simulink model "ball_and_beam"  (R2023b)
settings: Solver=VariableStepAuto  StartTime=0.0  StopTime=inf  RelTol=1e-3
values from neighbouring files (symbols this model uses):
  A = [0  1; 0  0]    [1-dof.mat]    (also in 2-dof.mat = [0 0 0 0 1 0 0 0 0 0 0 0 ... (16 elements, 4x4)]; ball_balancing_platform.mat = [0 0 0 0 0 0 0 0 0 0 0 0 ... (64 elements, 8x8)])
  B = [0 -0.1692]    [1-dof.mat]    (also in 2-dof.mat = [0  0; -0.253868468945  0; 0  0; 0  0.253868468945]; ball_balancing_platform.mat = [0 0 0 0 0 0 1 0 0 0 0 0 ... (16 elements, 8x2)])
  C = [1 0]    [1-dof.mat]    (also in 2-dof.mat = [1  0  0  0; 0  0  1  0]; ball_balancing_platform.mat = [1 0 0 0 0 1 0 0 0 0 1 0 ... (32 elements, 4x8)])
  D = 0    [1-dof.mat]    (also in 2-dof.mat = [0  0; 0  0]; ball_balancing_platform.mat = [0  0; 0  0; 0  0; 0  0])
libraries: robotlib x2, mpclib x1, aerolibanimutils x1
settings Model: Creator=farhan  LastModifiedBy=farhan

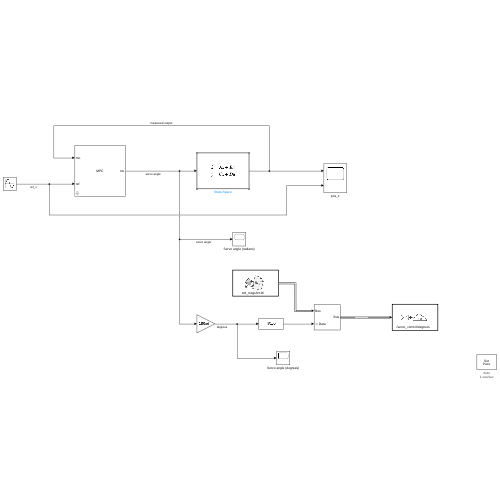
[thumbnail: Simulink's stored preview of the top-level diagram]
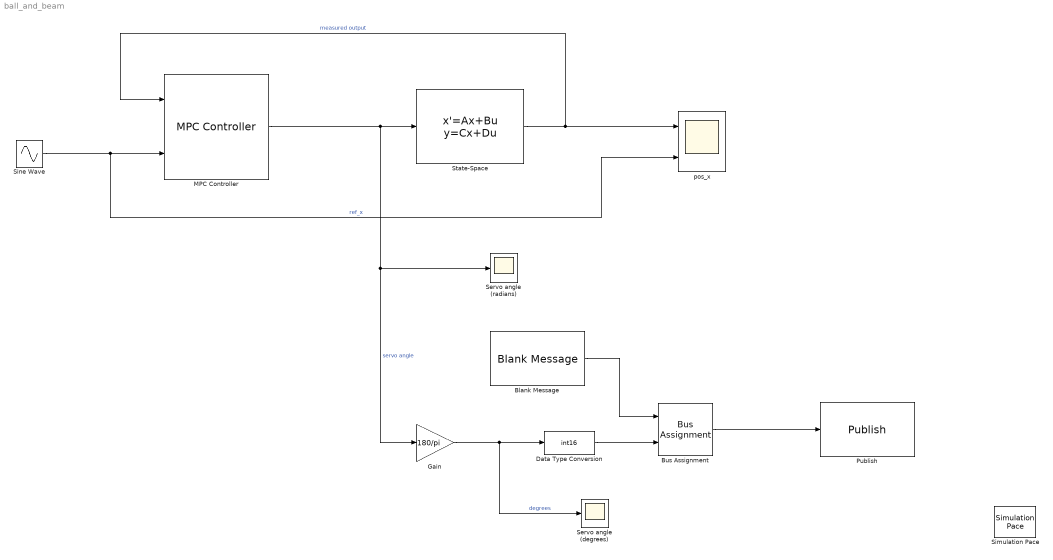
== system ball_and_beam ==
  Blank Message : robotlib/Blank Message  messageClass=Message  entityType=std_msgs/Int16  messageType=std_msgs/Int16  SampleTime=inf  legacyBusStruct=off
  Bus Assignment : BusAssignment  AssignedSignals=Data
  Data Type Conversion : DataTypeConversion  OutDataTypeStr=int16  SaturateOnIntegerOverflow=off  RndMeth=Floor
  Gain : Gain  Gain=180/pi
  MPC Controller : mpclib/MPC Controller  SCDEnableBlockLinearizationSpecification=on  mpcobj=mpc1  is_multiple=0  enable_value=0  return_u0=off  updateMPCinCallerWorkspace=on  md_inport=off  mv_inport=off  uref_inport=off  return_cost=off  return_mvseq=off  return_qpstatus=off  return_xseq=off  return_state=off  return_ovseq=off  state_inport=off  umin_inport=off  umax_inport=off  ymin_inport=off  ymax_inport=off  cc_inport=off  ywt_inport=off  uwt_inport=off  duwt_inport=off  rhoeps_inport=off  pm_inport=off  MaximumP=10  HorizonChoice=FixedHorizon  n_ts=0.1  n_p=6  n_mv=1  n_md=0  n_ud=0  n_mo=1  n_uo=0  BlockDataType=double  SampleTimeInherited=off  switch_inport=off
  Publish : robotlib/Publish  topicSource=Specify your own  topic=/servo_control/degrees  messageType=std_msgs/Int16  legacyBusStruct=off  messageQueueLength=1
  Servo angle (degrees) : Scope
  Servo angle (radians) : Scope
  Simulation Pace : aerolibanimutils/Simulation Pace  SimulationPace=1  SleepMode=Auto  OutputPaceError=off  SampleTime=1/30
  Sine Wave : Sin  Amplitude=0.15  Frequency=2*pi/6  SampleTime=0
  State-Space : StateSpace  A=A  B=B  C=C  D=D  InitialCondition=0
  pos_x : Scope  NumInputPorts=2
  wires:
  MPC Controller/1 -> Gain/1, Servo angle (radians)/1, State-Space/1  "servo angle"
  State-Space/1 -> MPC Controller/1, pos_x/1  "measured output"
  Sine Wave/1 -> pos_x/2, MPC Controller/2  "ref_x"
  Gain/1 -> Servo angle (degrees)/1, Data Type Conversion/1  "degrees"
  Blank Message/1 -> Bus Assignment/1
  Data Type Conversion/1 -> Bus Assignment/2
  Bus Assignment/1 -> Publish/1
